simulink model "Task3"  (R2020a)
settings: Solver=ode113  StartTime=0.0  StopTime=10000  MaxStep=1e-2  RelTol=1e-3
settings Model: Creator=dvdia  LastModifiedBy=dvdia
settings SFSimCC: CustomCodeUndefinedFunction=UseInterfaceOnly

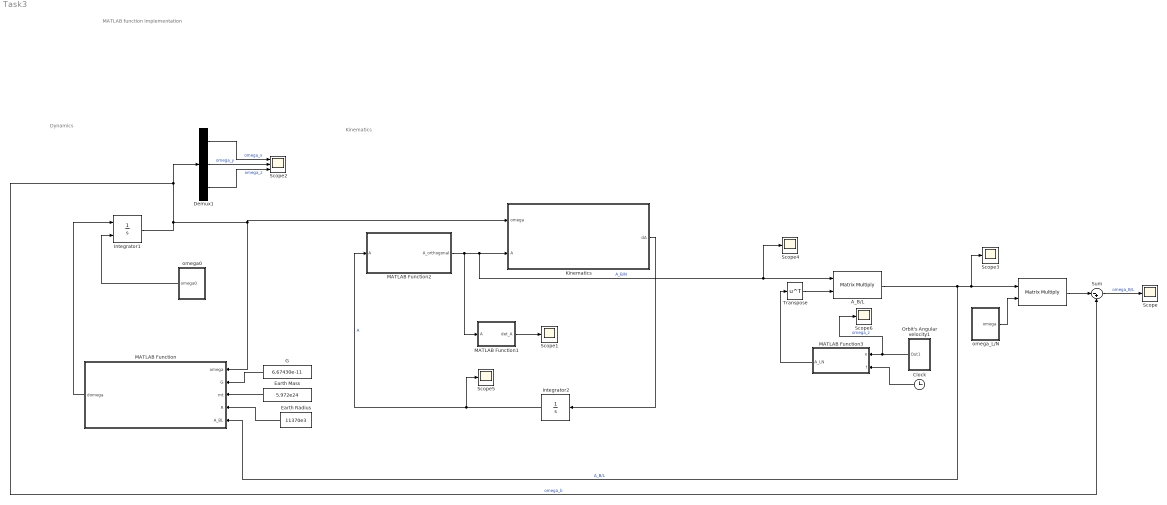
== system Task3 ==
  note: Kinematics
  note: Dynamics
  note: MATLAB function implementation
  " " : Product  Multiplication=Matrix(*)
  A_B/L : Product  Multiplication=Matrix(*)
  Clock : Clock
  Demux1 : Demux  Outputs=3
  Earth Mass : Constant  Value=5.972e24
  Earth Radius : Constant  Value=11370e3
  G : Constant  Value=6.67430e-11
  Integrator1 : Integrator  InitialConditionSource=external  InitialCondition=[ 0 0 5.972e24*6.67430e-11/(6371000^3)]
  Integrator2 : Integrator  InitialCondition=eye(3)
  Kinematics : MATLAB Function  TreatAsAtomicUnit=on
  MATLAB Function : MATLAB Function  TreatAsAtomicUnit=on
  MATLAB Function1 : MATLAB Function  TreatAsAtomicUnit=on
  MATLAB Function2 : MATLAB Function  TreatAsAtomicUnit=on
  MATLAB Function3 : MATLAB Function  TreatAsAtomicUnit=on
  Orbit's Angular velocity1 : Subsystem
  Scope{,1,3..6} (6 alike) : Scope
  Scope2 : Scope  NumInputPorts=3
  Sum : Sum  Inputs=|-+
  Transpose : Math  Operator=transpose  SignedPower=on  SaturateOnIntegerOverflow=on
  omega0 : Subsystem
  omega_L/N : Subsystem
  wires:
  Integrator2/1 -> Scope5/1, MATLAB Function2/1(A)  "A"
  Demux1/1 -> Scope2/1  "omega_x"
  MATLAB Function2/1(A_orthogonal) -> MATLAB Function1/1(A), Scope4/1, A_B/L/1, Kinematics/2(A)  "A_B/N"
  Demux1/2 -> Scope2/2  "omega_y"
  MATLAB Function/1(domega) -> Integrator1/1
  MATLAB Function1/1(det_A) -> Scope1/1
  Integrator1/1 -> Sum/2, Demux1/1, MATLAB Function/1(omega), Kinematics/1(omega)  "omega_b"
  Kinematics/1(dA) -> Integrator2/1
  Demux1/3 -> Scope2/3  "omega_z"
  Clock/1 -> MATLAB Function3/2(t)
  Orbit's Angular velocity1/1(Out1) -> Scope6/1, MATLAB Function3/1(n)  "omega_z"
  Transpose/1 -> A_B/L/2
  MATLAB Function3/1(A_LN) -> Transpose/1
  A_B/L/1 -> Scope3/1, " "/1, MATLAB Function/5(A_BL)  "A_B/L"
  omega0/1(omega0) -> Integrator1/2
  omega_L/N/1(omega) -> " "/2
  " "/1 -> Sum/1
  Sum/1 -> Scope/1  "omega_B/L"
  Earth Mass/1 -> MATLAB Function/3(mt)
  Earth Radius/1 -> MATLAB Function/4(R)
  G/1 -> MATLAB Function/2(G)

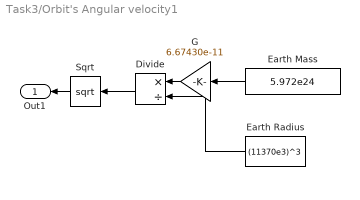
== system Task3/Orbit's Angular velocity1 ==
  Divide : Product  Inputs=*/
  Earth Mass : Constant  Value=5.972e24
  Earth Radius : Constant  Value=(11370e3)^3
  G : Gain  Gain=6.67430e-11
  Sqrt : Sqrt  SaturateOnIntegerOverflow=on
  Out1 : Outport
  wires:
  Earth Radius/1 -> Divide/2
  Divide/1 -> Sqrt/1
  Sqrt/1 -> Out1/1
  Earth Mass/1 -> G/1
  G/1 -> Divide/1

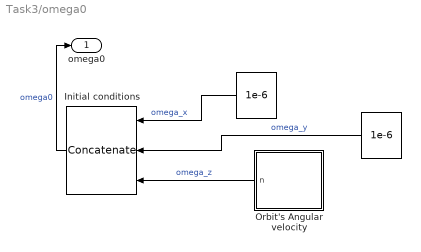
== system Task3/omega0 ==
  " " : Constant  Value=1e-6
  " " : Constant  Value=1e-6
  Initial conditions : Concatenate  NumInputs=3  ConcatenateDimension=3
  Orbit's Angular velocity : Subsystem
  omega0 : Outport
  wires:
  Orbit's Angular velocity/1(n) -> Initial conditions/3  "omega_z"
  Initial conditions/1 -> omega0/1  "omega0"
  " "/1 -> Initial conditions/1  "omega_x"
  " "/1 -> Initial conditions/2  "omega_y"

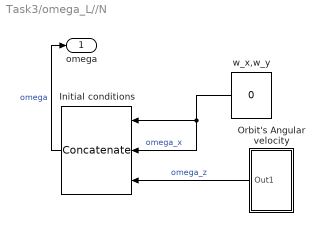
== system Task3/omega_L//N ==
  Initial conditions : Concatenate  NumInputs=3  ConcatenateDimension=3
  Orbit's Angular velocity : Subsystem
  w_x,w_y : Constant  Value=0
  omega : Outport
  wires:
  Orbit's Angular velocity/1(Out1) -> Initial conditions/3  "omega_z"
  Initial conditions/1 -> omega/1  "omega"
  w_x,w_y/1 -> Initial conditions/2, Initial conditions/1  "omega_x"

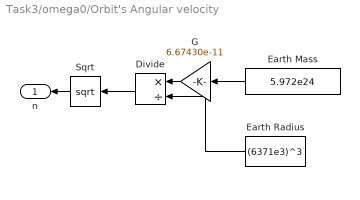
== system Task3/omega0/Orbit's Angular velocity ==
  Divide : Product  Inputs=*/
  Earth Mass : Constant  Value=5.972e24
  Earth Radius : Constant  Value=(6371e3)^3
  G : Gain  Gain=6.67430e-11
  Sqrt : Sqrt  SaturateOnIntegerOverflow=on
  n : Outport
  wires:
  G/1 -> Divide/1
  Earth Mass/1 -> G/1
  Sqrt/1 -> n/1
  Divide/1 -> Sqrt/1
  Earth Radius/1 -> Divide/2

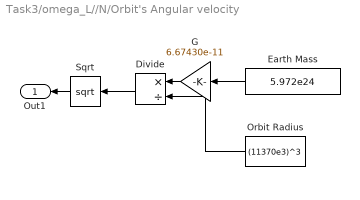
== system Task3/omega_L//N/Orbit's Angular velocity ==
  Divide : Product  Inputs=*/
  Earth Mass : Constant  Value=5.972e24
  G : Gain  Gain=6.67430e-11
  Orbit Radius : Constant  Value=(11370e3)^3
  Sqrt : Sqrt  SaturateOnIntegerOverflow=on
  Out1 : Outport
  wires:
  G/1 -> Divide/1
  Earth Mass/1 -> G/1
  Sqrt/1 -> Out1/1
  Divide/1 -> Sqrt/1
  Orbit Radius/1 -> Divide/2

== matlab function Task3/Kinematics ==
  data: omega input; dA output; A input
function dA = fcn(omega,A)


omega_x = omega(1);
omega_y = omega(2);
omega_z = omega(3);

w_cross = [ 0 -omega_z omega_y
            omega_z 0 -omega_x
            -omega_y omega_x 0 ];
        
dA = - w_cross * A ;
end

== matlab function Task3/MATLAB Function ==
  data: omega input; domega output; G input; mt input; R input; A_BL input
function domega = fcn(omega,G,mt,R,A_BL)

% Inertia moments


I_x = 0.01;         %  [kg*m^2]
% I_x = 0.05;         %  [kg*m^2]
I_y = 0.05;       %  [kg*m^2]
% I_y = 0.09;       %  [kg*m^2]
I_z = 0.09;       %  [kg*m^2]
% I_z = 0.01;       %  [kg*m^2]


% Set omegas
omega_x = omega(1);
omega_y = omega(2);
omega_z = omega(3);

% Calculate coefficients

c = A_BL * [1;0;0];

% Compute d_omegas with gravity gradient torque

domega_x = (I_y-I_z)*omega_y*omega_z/I_x  + 3*G*mt/R^3/I_x * (I_z - I_y) *c(3)*c(2);
domega_y = (I_z-I_x)*omega_x*omega_z/I_y  + 3*G*mt/R^3/I_y * (I_x - I_z) *c(1)*c(3);
domega_z = (I_x - I_y)*omega_y*omega_x / I_z  + 3*G*mt/R^3/I_z * (I_y - I_x) *c(2)*c(1);

domega = [ domega_x domega_y domega_z ];
end

== matlab function Task3/MATLAB Function1 ==
  data: A input; det_A output
function det_A = fcn(A)

det_A = det(A);

== matlab function Task3/MATLAB Function2 ==
  data: A input; A_orthogonal output
function A_orthogonal = orthonormalizer(A)

% Iterative formulas for orthonormalization
% first order approximation: single step iteration
A_orthogonal = A*3/2 - A*(A')*A/2;

end

== matlab function Task3/MATLAB Function3 ==
  data: n input; A_LN output; t input
function A_LN = matrixA_LN(n,t)

A_LN = [cos(n*t)    sin(n*t)    0
        -sin(n*t)   cos(n*t)    0
        0           0           1];
end
